simulink model "ProblemStatewithRL"  (R2025b)
settings: Solver=VariableStepAuto  StartTime=0.0  StopTime=100  RelTol=1e-3
values from neighbouring files (symbols this model uses):
  case_id = cases(i)    [evaluate_all_disturbances.m]    (also in run_trained_agent.m = 5; train_sac.m = curriculumCases(stage); train_sac_5.m = 5)
libraries: slpidlib x1, rllib x1
settings Model: Creator=goelp4  LastModifiedBy=Hp
settings OptimizationCC: BlockReduction=off  DefaultParameterBehavior=Inlined  BufferReuse=off
settings DebuggingCC: UnconnectedInputMsg=warning  UnconnectedOutputMsg=warning  UnconnectedLineMsg=warning
settings ModelReferenceCC: EnableRefExpFcnMdlSchedulingChecks=on
settings RTWCC: GPUComputeCapability=3.5  DLArmComputeVersion=19.05

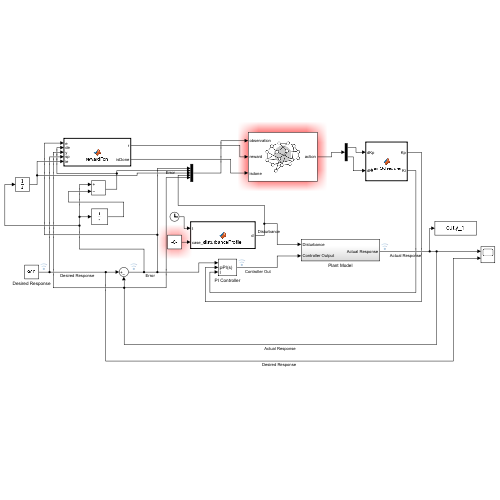
[thumbnail: Simulink's stored preview of the top-level diagram]
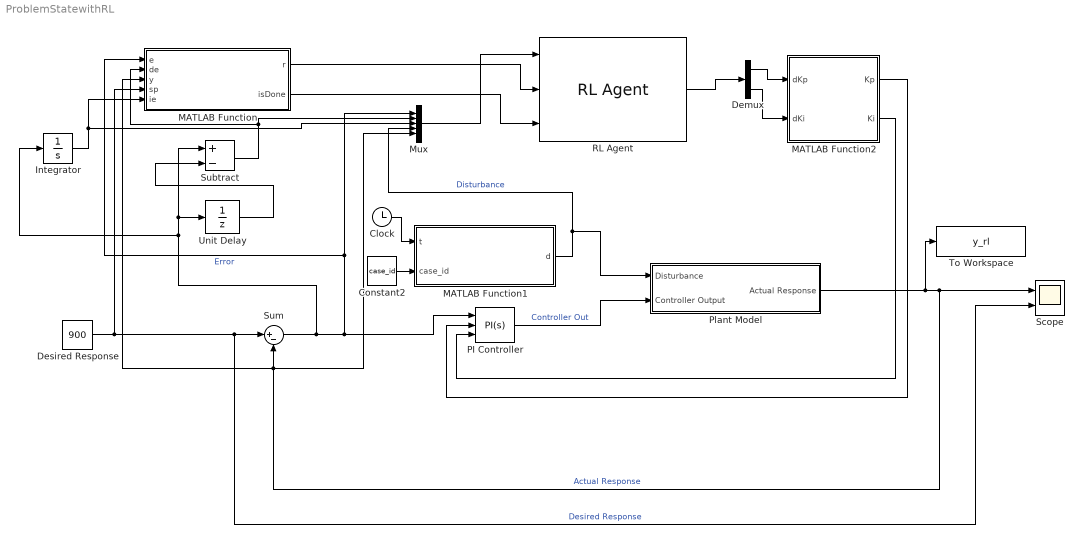
== system ProblemStatewithRL ==
  Clock : Clock
  Constant2 : Constant  Value=case_id
  Demux : Demux  Outputs=2
  Desired Response : Constant  Value=900
  Integrator : Integrator
  MATLAB Function : MATLAB Function  TreatAsAtomicUnit=on
  MATLAB Function1 : MATLAB Function  TreatAsAtomicUnit=on
  MATLAB Function2 : MATLAB Function  TreatAsAtomicUnit=on
  Mux : Mux  Inputs=5
  PI Controller : slpidlib/PID Controller  Controller=PI  Form=Parallel  TimeDomain=Continuous-time  UseExternalTs=off  SampleTime=-1  IntegratorMethod=Forward Euler  FilterMethod=Forward Euler  ControllerParametersSource=external  P=1  I=1  UseKiTs=off  D=0  UseExternalDerivativeSource=off  N=100  UseFilter=on  TunerSelectOption=Transfer Function Based (PID Tuner App)  InitialConditionSource=internal  InitialConditionForIntegrator=0  InitialConditionForFilter=0  DifferentiatorICPrevScaledInput=0  ExternalReset=none  TrackingMode=off  Kt=1  LimitOutput=off  SatLimitsSource=internal  UpperSaturationLimit=inf  LowerSaturationLimit=-inf  LinearizeAsGain=on  AntiWindupMode=none  Kb=1  LimitIntegrator=off  UpperIntegratorSaturationLimit=inf  LowerIntegratorSaturationLimit=-inf  POutMin=[]  POutMax=[]  IOutMin=[]  IOutMax=[]  DOutMin=[]  DOutMax=[]  NOutMin=[]  NOutMax=[]  SumOutMin=[]  SumOutMax=[]  SaturationOutMin=[]  SaturationOutMax=[]  PParamMin=[]  PParamMax=[]  IParamMin=[]  IParamMax=[]  DParamMin=[]  DParamMax=[]  NParamMin=[]  NParamMax=[]  KbParamMin=[]  KbParamMax=[]  KtParamMin=[]  KtParamMax=[]  KbOutMin=[]  KbOutMax=[]  KtOutMin=[]  KtOutMax=[]  IntegratorOutMin=[]  IntegratorOutMax=[]  FilterOutMin=[]  FilterOutMax=[]  SumI1OutMin=[]  SumI1OutMax=[]  SumI2OutMin=[]  SumI2OutMax=[]  SumI3OutMin=[]  SumI3OutMax=[]  SumI4OutMin=[]  SumI4OutMax=[]  SumDOutMin=[]  SumDOutMax=[]  DifferentiatorOutMin=[]  DifferentiatorOutMax=[]  FilterDiffOutCoefMin=[]  FilterDiffOutCoefMax=[]  ReciprocalOutMin=[]  ReciprocalOutMax=[]  SumDenOutMin=[]  SumDenOutMax=[]  SumNumOutMin=[]  SumNumOutMax=[]  DivideOutMin=[]  DivideOutMax=[]  UdiffTsProdOutMin=[]  UdiffTsProdOutMax=[]  NTsProdOutMin=[]  NTsProdOutMax=[]  UintegralTsProdOutMin=[]  UintegralTsProdOutMax=[]  UngainTsProdOutMin=[]  UngainTsProdOutMax=[]  ClampingZeroOutDataTypeStr=Inherit: Inherit via back propagation  ClampingZeroOutMin=[]  ClampingZeroOutMax=[]  FilterDenConstantOutDataTypeStr=Inherit: Inherit via back propagation  FilterDenConstantOutMin=[]  FilterDenConstantOutMax=[]  PCopyOutDataTypeStr=Inherit: Inherit via back propagation  PCopyOutMin=[]  PCopyOutMax=[]  NCopyOutDataTypeStr=Inherit: Inherit via back propagation  NCopyOutMin=[]  NCopyOutMax=[]  IntegratorContinuousStateAttributes=''  IntegratorStateMustResolveToSignalObject=off  IntegratorRTWStateStorageClass=Auto  FilterContinuousStateAttributes=''  FilterStateMustResolveToSignalObject=off  FilterRTWStateStorageClass=Auto  ParallelPVariant=ExternalParameters  IdealPVariant=Disabled  IVariant=ExternalParameters  DVariant=Disabled  IntegratorVariant=Continuous  SatVariant=Disabled  AWVariant=Passthrough  PCopyVariant=Disabled  TRVariant=Disabled  FdbkBlocksVariant=Forward  IdealPFdbkVariant=Disabled  SatFdbkVariant=Disabled  DerivativeFilterVariant=Disabled  NVariant=Disabled  NCopyVariant=Disabled_SignalSpec  FilterICVariant=Disabled  IntegratorICVariant=InternalICs  ExternalResetVariant=Disabled  TRSumVariant=Passthrough  SumFdbkVariant=Disabled  SumVariant=Sum_PI  TsampFilterVariant=InternalTs  TsampNgainVariant=Passthrough  TsampIntegralVariant=Disabled_SignalSpec  ExternalSaturationOutDataTypeStr=Inherit: Same as second input  DerivativeSourceVariant=Disabled  PreIntVariant=InternalPreInt
  Plant Model : Subsystem
  RL Agent : rllib/RL Agent  Agent=agentObj  ExternalActionAsInput=off  ProvideLastAction=off  ProvideCumRwd=off  TreatAsDirectFeedthrough=on  UseStrictObservationDataTypes=off
  Scope : Scope  NumInputPorts=2
      settings: ActiveDisplayYMinimum=-108.61281564041542  ActiveDisplayYMaximum=1322.9375622322832
  Subtract : Sum  Inputs=+-
  Sum : Sum  Inputs=|+-
  To Workspace : ToWorkspace  VariableName=y_rl  SampleTime=-1
  Unit Delay : UnitDelay  SampleTime=-1  HasFrameUpgradeWarning=on
  wires:
  Desired Response/1 -> MATLAB Function/4(sp), Sum/1, Scope/2  "Desired Response"
  Plant Model/1(Actual Response) -> To Workspace/1, Mux/5, MATLAB Function/3(y), Sum/2, Scope/1  "Actual Response"
  PI Controller/1 -> Plant Model/2(Controller Output)  "Controller Out"
  Sum/1 -> Integrator/1, Subtract/1, Unit Delay/1, Mux/1, MATLAB Function/1(e), PI Controller/1  "Error"
  MATLAB Function1/1(d) -> Mux/4, Plant Model/1(Disturbance)  "Disturbance"
  Mux/1 -> RL Agent/1
  RL Agent/1 -> Demux/1
  MATLAB Function2/2(Ki) -> PI Controller/3
  MATLAB Function2/1(Kp) -> PI Controller/2
  MATLAB Function/1(r) -> RL Agent/2
  Unit Delay/1 -> Subtract/2
  MATLAB Function/2(isDone) -> RL Agent/3
  Subtract/1 -> Mux/2, MATLAB Function/2(de)
  Integrator/1 -> Mux/3, MATLAB Function/5(ie)
  Constant2/1 -> MATLAB Function1/2(case_id)
  Clock/1 -> MATLAB Function1/1(t)
  Demux/1 -> MATLAB Function2/1(dKp)
  Demux/2 -> MATLAB Function2/2(dKi)

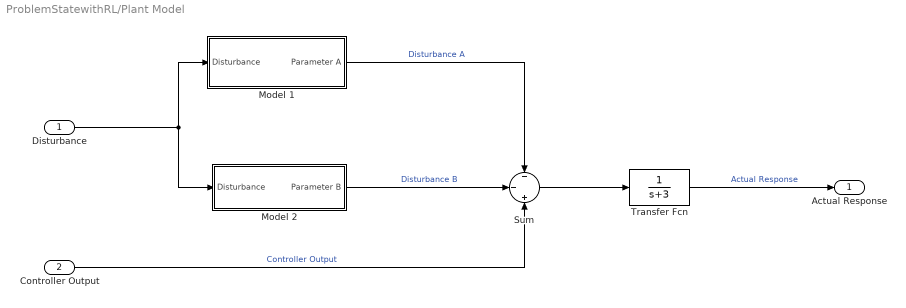
== system ProblemStatewithRL/Plant Model ==
  Disturbance : Inport
  Controller Output : Inport  Port=2
  Model 1 : Subsystem
  Model 2 : Subsystem
  Sum : Sum  Inputs=-|-|+
  Transfer Fcn : TransferFcn  Denominator=[1 3]
  Actual Response : Outport
  wires:
  Transfer Fcn/1 -> Actual Response/1  "Actual Response"
  Sum/1 -> Transfer Fcn/1
  Disturbance/1 -> Model 2/1(Disturbance), Model 1/1(Disturbance)
  Controller Output/1 -> Sum/3  "Controller Output"
  Model 2/1(Parameter B) -> Sum/2  "Disturbance B"
  Model 1/1(Parameter A) -> Sum/1  "Disturbance A"

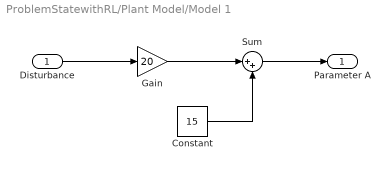
== system ProblemStatewithRL/Plant Model/Model 1 ==
  Disturbance : Inport
  Constant : Constant  Value=15
  Gain : Gain  Gain=20
  Sum : Sum  Inputs=|++
  Parameter A : Outport
  wires:
  Disturbance/1 -> Gain/1
  Gain/1 -> Sum/1
  Sum/1 -> Parameter A/1
  Constant/1 -> Sum/2

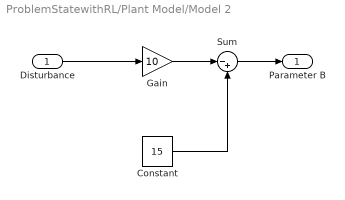
== system ProblemStatewithRL/Plant Model/Model 2 ==
  Disturbance : Inport
  Constant : Constant  Value=15
  Gain : Gain  Gain=10
  Sum : Sum  Inputs=|-+
  Parameter B : Outport
  wires:
  Disturbance/1 -> Gain/1
  Gain/1 -> Sum/1
  Sum/1 -> Parameter B/1
  Constant/1 -> Sum/2

== matlab function ProblemStatewithRL/MATLAB Function1 ==
  data: t input; d output; case_id input
function d = disturbanceProfile(t, case_id)

%% ==================================================
% PREALLOCATE
%% ==================================================
timeVec = zeros(1,21);
distVec = zeros(1,21);

%% ==================================================
% SELECT PROFILE
%% ==================================================
switch case_id

    %% ================= 5% =================
    case 5

        timeVec = 0:50:1000;

        distVec = [...
            0.00 0.05 0.10 0.15 0.20 ...
            0.25 0.30 0.35 0.40 0.45 ...
            0.50 0.45 0.40 0.35 0.30 ...
            0.25 0.20 0.15 0.10 0.05 0.00];

    %% ================= 10% =================
    case 10

        timeVec = 0:100:1000;

        distVec = [...
            0.0 0.1 0.2 0.3 0.4 ...
            0.5 0.4 0.3 0.2 0.1 0.0];

    %% ================= 15% =================
    case 15

        timeVec = 0:100:1000;

        distVec = [...
            0.0 0.15 0.30 0.45 0.60 ...
            0.75 0.60 0.45 0.30 0.15 0.0];

    %% ================= 20% =================
    case 20

        timeVec = 0:100:1000;

        distVec = [...
            0.0 0.2 0.4 0.6 0.8 ...
            1.0 0.8 0.6 0.4 0.2 0.0];

    %% ================= 30% =================
    case 30

        timeVec = [0 150 300 450 600 750 900 1000];

        distVec = [...
            0.0 0.3 0.6 0.9 ...
            0.6 0.3 0.0 0.0];

    %% ================= LARGE STEP =================
    case 99

        timeVec = [0 400 401 1000];

        distVec = [0.9 0.9 0.2 0.2];

end

%% ==================================================
% STEPWISE LOOKUP
%% ==================================================
d = distVec(1);

for k = 1:length(timeVec)-1

    if t >= timeVec(k) && t < timeVec(k+1)

        d = distVec(k);
        break;

    end

end

== matlab function ProblemStatewithRL/MATLAB Function ==
  data: e input; r output; de input; y input; sp input; ie input; isDone output
function [r, isDone] = rewardFcn(e, de, y, sp, ie)

%% NORMALIZATION
e_n = e/sp;

de_n = de/sp;

%% =====================================================
% 1. MAIN ERROR
%% =====================================================
R1 = -10*abs(e_n);

%% =====================================================
% 2. APPROACH VELOCITY
% MOST IMPORTANT TERM
%% =====================================================
R2 = -20*de_n*sign(e_n);

%% =====================================================
% 3. FAST CLOSE BONUS
%% =====================================================
if abs(e_n) < 0.05

    R3 = +80;

else

    R3 = 0;

end

%% =====================================================
% 4. OVERSHOOT ALLOWED
%% =====================================================
if y > 1.6*sp

    OS = (y-sp)/sp;

    R4 = -2*OS^2;

else

    R4 = 0;

end

%% =====================================================
% 5. UNDERSHOOT PENALTY
%% =====================================================
if y < 0.7*sp

    US = (sp-y)/sp;

    R5 = -20*US^2;

else

    R5 = 0;

end

%% =====================================================
% 6. FINAL PRECISION
%% =====================================================
if abs(e_n) < 0.01

    R6 = +150;

else

    R6 = 0;

end

%% =====================================================
% 7. INSTABILITY
%% =====================================================
if abs(y) > 2.5*sp

    R7 = -5000;

    isDone = 1;

else

    R7 = 0;

    isDone = 0;

end

%% FINAL
r = R1 + R2 + R3 + ...
    R4 + R5 + R6 + R7;

end

== matlab function ProblemStatewithRL/MATLAB Function2 ==
  data: dKp input; Kp output; Ki output; dKi input
function [Kp, Ki] = gainScheduler(dKp, dKi)

%% =====================================================
% BASE PI

Kp_base = 90;
Ki_base = 40;

Kp = Kp_base + 40*dKp;

Ki = Ki_base + 20*dKi;

%% =====================================================
% LIMITS
%% =====================================================


end
